simulink model "cruise_control_dut_harness"  (R2014b)
settings: Solver=FixedStepDiscrete  StartTime=0  StopTime=0.029999999999999999  FixedStep=0.01  RelTol=1e-3
undefined symbols (not defined in the file): sigbuilder_block
libraries: simulink x1
settings Model: SldvGeneratedHarnessModel=TestUnitModel=cosim_cruise_control|  RecordCoverage=on  CovMetricSettings=dcmoeb  CovHTMLOptions=-aTS=1 -bRG=1 -bTC=0 -hTR=0 -nFC=0 -scm=1 -bcm=1  covSaveCumulativeToWorkspaceVar=off  CovSaveSingleToWorkspaceVar=off  CovReportOnPause=off  CovModelRefEnable=off  CovExternalEMLEnable=on  Creator=The MathWorks Inc.  LastModifiedBy=kotsuka
settings DataIOCC: SaveFormat=StructureWithTime  SignalLoggingSaveFormat=ModelDataLogs
settings OptimizationCC: BlockReduction=off  ConditionallyExecuteInputs=off  InlineParams=on  InlineInvariantSignals=on  ExpressionFolding=off  ExpressionDepthLimit=2147483647  InitFltsAndDblsToZero=on  EfficientMapNaN2IntZero=off
settings DebuggingCC: SaveWithParameterizedLinksMsg=none  UnderspecifiedInitializationDetection=Classic  MergeDetectMultiDrivingBlocksExec=none  SignalResolutionControl=TryResolveAllWithWarning  InheritedTsInSrcMsg=none  FcnCallInpInsideContextMsg=UseLocalSettings  StateNameClashWarn=warning
settings GRTTargetCC: TargetFcnLib=ansi_tfl_tmw.mat  CombineOutputUpdateFcns=off  GRTInterface=on
settings ConfigComp: Description=Design Verifier Custom Configuration Component  DVMaxProcessTime=60  DVMakeOutputFilesUnique=off  DVParameters=on  DVModelCoverageObjectives=MCDC  DVMaxTestCaseSteps=500  DVTestSuiteOptimization=CombinedObjectives  DVAssertions=EnableAll  DVProofAssumptions=EnableAll  DVCovFilter=on  DVDetectActiveLogic=on  DVProvingStrategy=FindViolation

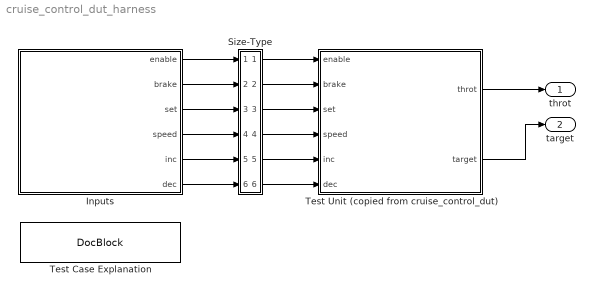
== system cruise_control_dut_harness ==
  Inputs : Subsystem  Tag=STV Subsys  LoadFcn=sigbuilder_block('load');  StartFcn=sigbuilder_block('start');  StopFcn=sigbuilder_block('stop');  ClipboardFcn=sigbuilder_block('clipboard');  mask(Sigbuilder block){}
      mask init:
      | if ~strcmp(get_param(bdroot(gcb),'SimulationStatus'),'stopped'),tuvar = sigbuilder_block('maskInit'); end
      settings: CopyFcn=sigbuilder_block('copy');  DeleteFcn=sigbuilder_block('delete');  ModelCloseFcn=sigbuilder_block('modelClose');  PreSaveFcn=sigbuilder_block('preSave');  PauseFcn=sigbuilder_block('pause');  ContinueFcn=sigbuilder_block('continue');  NameChangeFcn=sigbuilder_block('namechange');  OpenFcn=sigbuilder_block('open');  CloseFcn=sigbuilder_block('close');
      mask Display: plot(0, 0, 100, 100,[2, 2, 32, 32, 2], [68, 8, 8, 68, 68],[32, 2], [38, 38], [32, 19, 2],[53, 60, 44], [32, 17, 17, 2],[16, 16, 31, 31]);txt = getActiveGroup(gcbh);text(2, 100, txt,'verticalAlignment', 'top');
  Size-Type : Subsystem
  Test Case Explanation : simulink/Model-Wide Utilities/DocBlock  DocumentType=Text
  Test Unit (copied from cruise_control_dut) : Subsystem
  throt : Outport
  target : Outport  Port=2
  wires:
  Inputs/1(enable) -> Size-Type/1(In1)
  Size-Type/1(Out1) -> Test Unit (copied from cruise_control_dut)/1(enable)
  Inputs/2(brake) -> Size-Type/2(In2)
  Size-Type/2(Out2) -> Test Unit (copied from cruise_control_dut)/2(brake)
  Inputs/3(set) -> Size-Type/3(In3)
  Size-Type/3(Out3) -> Test Unit (copied from cruise_control_dut)/3(set)
  Inputs/4(speed) -> Size-Type/4(In4)
  Size-Type/4(Out4) -> Test Unit (copied from cruise_control_dut)/4(speed)
  Inputs/5(inc) -> Size-Type/5(In5)
  Size-Type/5(Out5) -> Test Unit (copied from cruise_control_dut)/5(inc)
  Inputs/6(dec) -> Size-Type/6(In6)
  Size-Type/6(Out6) -> Test Unit (copied from cruise_control_dut)/6(dec)
  Test Unit (copied from cruise_control_dut)/1(throt) -> throt/1
  Test Unit (copied from cruise_control_dut)/2(target) -> target/1

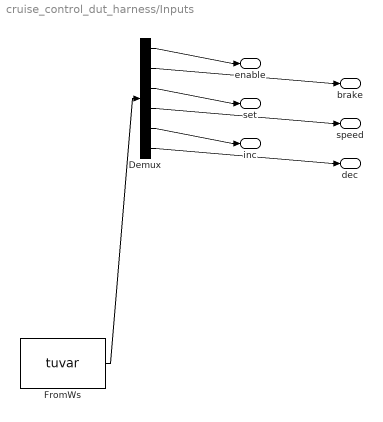
== system cruise_control_dut_harness/Inputs ==
  Demux : Demux  Tag=STV Demux  Outputs=6
  FromWs : FromWorkspace  Tag=STV FromWs  VariableName=tuvar  SampleTime=0
      SigBuilderData=|
      | dataSet(1).timeRange = [0 0.01]
      | dataSet(1).name = 'テスト ケース 1'
      | dataSet(2).timeRange = [0 0.01]
      | dataSet(2).name = 'テスト ケース 2'
      | dataSet(3).timeRange = [0 0.01]
      | dataSet(3).name = 'テスト ケース 3'
      | dataSet(4).timeRange = [0 0.01]
      | dataSet(4).name = 'テスト ケース 4'
      | dataSet(5).timeRange = [0 0.01]
      | dataSet(5).name = 'テスト ケース 5'
      | dataSet(6).timeRange = [0 0.01]
      | dataSet(6).name = 'テスト ケース 6'
      | dataSet(7).timeRange = [0 0.02]
      | dataSet(7).name = 'テスト ケース 7'
      | dataSet(8).timeRange = [0 0.03]
      | dataSet(8).name = 'テスト ケース 8'
      | dataSet(9).timeRange = [0 0.03]
      | dataSet(9).name = 'テスト ケース 9'
      | sbobj.Name = 'Signal Builder'
      | sbobj.Groups(1).Name = 'テスト ケース 1'
      | sbobj.Groups(1).Signals(1).Name = 'enable'
      | sbobj.Groups(1).Signals(1).XData = [0 0.01]
      | sbobj.Groups(1).Signals(1).YData = [0 0]
      | sbobj.Groups(1).Signals(2).Name = 'brake'
      | sbobj.Groups(1).Signals(2).XData = [0 0.01]
      | sbobj.Groups(1).Signals(2).YData = [0 0]
      | sbobj.Groups(1).Signals(3).Name = 'set'
      | sbobj.Groups(1).Signals(3).XData = [0 0.01]
      | sbobj.Groups(1).Signals(3).YData = [1 1]
      | sbobj.Groups(1).Signals(4).Name = 'speed'
      | sbobj.Groups(1).Signals(4).XData = [0 0.01]
      | sbobj.Groups(1).Signals(4).YData = [0 0]
      | sbobj.Groups(1).Signals(5).Name = 'inc'
      | sbobj.Groups(1).Signals(5).XData = [0 0.01]
      | sbobj.Groups(1).Signals(5).YData = [0 0]
      | sbobj.Groups(1).Signals(6).Name = 'dec'
      | sbobj.Groups(1).Signals(6).XData = [0 0.01]
      | sbobj.Groups(1).Signals(6).YData = [0 0]
      | sbobj.Groups(1).TimeRange = [0 0.01]
      | sbobj.Groups(2).Name = 'テスト ケース 2'
      | sbobj.Groups(2).Signals(1).Name = 'enable'
      | sbobj.Groups(2).Signals(1).XData = [0 0.01]
      | sbobj.Groups(2).Signals(1).YData = [1 1]
      | sbobj.Groups(2).Signals(2).Name = 'brake'
      | sbobj.Groups(2).Signals(2).XData = [0 0.01]
      | sbobj.Groups(2).Signals(2).YData = [1 1]
      | sbobj.Groups(2).Signals(3).Name = 'set'
      | sbobj.Groups(2).Signals(3).XData = [0 0.01]
      | sbobj.Groups(2).Signals(3).YData = [1 1]
      | sbobj.Groups(2).Signals(4).Name = 'speed'
      | sbobj.Groups(2).Signals(4).XData = [0 0.01]
      | sbobj.Groups(2).Signals(4).YData = [0 0]
      | sbobj.Groups(2).Signals(5).Name = 'inc'
      | sbobj.Groups(2).Signals(5).XData = [0 0.01]
      | sbobj.Groups(2).Signals(5).YData = [0 0]
      | sbobj.Groups(2).Signals(6).Name = 'dec'
      | sbobj.Groups(2).Signals(6).XData = [0 0.01]
      | sbobj.Groups(2).Signals(6).YData = [0 0]
      | sbobj.Groups(2).TimeRange = [0 0.01]
      | sbobj.Groups(3).Name = 'テスト ケース 3'
      | sbobj.Groups(3).Signals(1).Name = 'enable'
      | sbobj.Groups(3).Signals(1).XData = [0 0.01]
      | sbobj.Groups(3).Signals(1).YData = [0 0]
      | sbobj.Groups(3).Signals(2).Name = 'brake'
      | sbobj.Groups(3).Signals(2).XData = [0 0.01]
      | sbobj.Groups(3).Signals(2).YData = [0 0]
      | sbobj.Groups(3).Signals(3).Name = 'set'
      | sbobj.Groups(3).Signals(3).XData = [0 0.01]
      | sbobj.Groups(3).Signals(3).YData = [0 0]
      | sbobj.Groups(3).Signals(4).Name = 'speed'
      | sbobj.Groups(3).Signals(4).XData = [0 0.01]
      | sbobj.Groups(3).Signals(4).YData = [0 0]
      | sbobj.Groups(3).Signals(5).Name = 'inc'
      | sbobj.Groups(3).Signals(5).XData = [0 0.01]
      | sbobj.Groups(3).Signals(5).YData = [1 1]
      | sbobj.Groups(3).Signals(6).Name = 'dec'
      | sbobj.Groups(3).Signals(6).XData = [0 0.01]
      | sbobj.Groups(3).Signals(6).YData = [0 0]
      | sbobj.Groups(3).TimeRange = [0 0.01]
      | sbobj.Groups(4).Name = 'テスト ケース 4'
      | sbobj.Groups(4).Signals(1).Name = 'enable'
      | sbobj.Groups(4).Signals(1).XData = [0 0.01]
      | sbobj.Groups(4).Signals(1).YData = [1 1]
      | sbobj.Groups(4).Signals(2).Name = 'brake'
      | sbobj.Groups(4).Signals(2).XData = [0 0.01]
      | sbobj.Groups(4).Signals(2).YData = [0 0]
      | sbobj.Groups(4).Signals(3).Name = 'set'
      | sbobj.Groups(4).Signals(3).XData = [0 0.01]
      | sbobj.Groups(4).Signals(3).YData = [0 0]
      | sbobj.Groups(4).Signals(4).Name = 'speed'
      | sbobj.Groups(4).Signals(4).XData = [0 0.01]
      | sbobj.Groups(4).Signals(4).YData = [0 0]
      | sbobj.Groups(4).Signals(5).Name = 'inc'
      | sbobj.Groups(4).Signals(5).XData = [0 0.01]
      | sbobj.Groups(4).Signals(5).YData = [1 1]
      | sbobj.Groups(4).Signals(6).Name = 'dec'
      | sbobj.Groups(4).Signals(6).XData = [0 0.01]
      | sbobj.Groups(4).Signals(6).YData = [0 0]
      | sbobj.Groups(4).TimeRange = [0 0.01]
      | sbobj.Groups(5).Name = 'テスト ケース 5'
      | sbobj.Groups(5).Signals(1).Name = 'enable'
      | sbobj.Groups(5).Signals(1).XData = [0 0.01]
      | sbobj.Groups(5).Signals(1).YData = [1 1]
      | sbobj.Groups(5).Signals(2).Name = 'brake'
      | sbobj.Groups(5).Signals(2).XData = [0 0.01]
      | sbobj.Groups(5).Signals(2).YData = [0 0]
      | sbobj.Groups(5).Signals(3).Name = 'set'
      | sbobj.Groups(5).Signals(3).XData = [0 0.01]
      | sbobj.Groups(5).Signals(3).YData = [1 1]
      | sbobj.Groups(5).Signals(4).Name = 'speed'
      | sbobj.Groups(5).Signals(4).XData = [0 0.01]
      | sbobj.Groups(5).Signals(4).YData = [0 0]
      | sbobj.Groups(5).Signals(5).Name = 'inc'
      | sbobj.Groups(5).Signals(5).XData = [0 0.01]
      | sbobj.Groups(5).Signals(5).YData = [0 0]
      | sbobj.Groups(5).Signals(6).Name = 'dec'
      | sbobj.Groups(5).Signals(6).XData = [0 0.01]
      | sbobj.Groups(5).Signals(6).YData = [0 0]
      | sbobj.Groups(5).TimeRange = [0 0.01]
      | sbobj.Groups(6).Name = 'テスト ケース 6'
      | sbobj.Groups(6).Signals(1).Name = 'enable'
      | sbobj.Groups(6).Signals(1).XData = [0 0.01]
      | sbobj.Groups(6).Signals(1).YData = [0 0]
      | sbobj.Groups(6).Signals(2).Name = 'brake'
      | sbobj.Groups(6).Signals(2).XData = [0 0.01]
      | sbobj.Groups(6).Signals(2).YData = [0 0]
      | sbobj.Groups(6).Signals(3).Name = 'set'
      | sbobj.Groups(6).Signals(3).XData = [0 0.01]
      | sbobj.Groups(6).Signals(3).YData = [1 1]
      | sbobj.Groups(6).Signals(4).Name = 'speed'
      | sbobj.Groups(6).Signals(4).XData = [0 0.01]
      | sbobj.Groups(6).Signals(4).YData = [0 0]
      | sbobj.Groups(6).Signals(5).Name = 'inc'
      | sbobj.Groups(6).Signals(5).XData = [0 0.01]
      | sbobj.Groups(6).Signals(5).YData = [0 0]
      | sbobj.Groups(6).Signals(6).Name = 'dec'
      | sbobj.Groups(6).Signals(6).XData = [0 0.01]
      | sbobj.Groups(6).Signals(6).YData = [1 1]
      | sbobj.Groups(6).TimeRange = [0 0.01]
      | sbobj.Groups(7).Name = 'テスト ケース 7'
      | sbobj.Groups(7).Signals(1).Name = 'enable'
      | sbobj.Groups(7).Signals(1).XData = [0 0.01 0.02]
      | sbobj.Groups(7).Signals(1).YData = [1 1 1]
      | sbobj.Groups(7).Signals(2).Name = 'brake'
      | sbobj.Groups(7).Signals(2).XData = [0 0.01 0.02]
      | sbobj.Groups(7).Signals(2).YData = [0 0 0]
      | sbobj.Groups(7).Signals(3).Name = 'set'
      | sbobj.Groups(7).Signals(3).XData = [0 0.01 0.01 0.02]
      | sbobj.Groups(7).Signals(3).YData = [1 1 0 0]
      | sbobj.Groups(7).Signals(4).Name = 'speed'
      | sbobj.Groups(7).Signals(4).XData = [0 0.01 0.02]
      | sbobj.Groups(7).Signals(4).YData = [0 0 0]
      | sbobj.Groups(7).Signals(5).Name = 'inc'
      | sbobj.Groups(7).Signals(5).XData = [0 0.01 0.01 0.02]
      | sbobj.Groups(7).Signals(5).YData = [1 1 0 0]
      | sbobj.Groups(7).Signals(6).Name = 'dec'
      | sbobj.Groups(7).Signals(6).XData = [0 0.01 0.02]
      | sbobj.Groups(7).Signals(6).YData = [0 0 0]
      | sbobj.Groups(7).TimeRange = [0 0.02]
      | sbobj.Groups(8).Name = 'テスト ケース 8'
      | sbobj.Groups(8).Signals(1).Name = 'enable'
      | sbobj.Groups(8).Signals(1).XData = [0 0.01 0.02 0.03]
      | sbobj.Groups(8).Signals(1).YData = [1 1 1 1]
      | sbobj.Groups(8).Signals(2).Name = 'brake'
      | sbobj.Groups(8).Signals(2).XData = [0 0.01 0.02 0.03]
      | sbobj.Groups(8).Signals(2).YData = [0 0 0 0]
      | sbobj.Groups(8).Signals(3).Name = 'set'
      | sbobj.Groups(8).Signals(3).XData = [0 0.01 0.01 0.02 0.02 0.03]
      | sbobj.Groups(8).Signals(3).YData = [1 1 0 0 1 1]
      | sbobj.Groups(8).Signals(4).Name = 'speed'
      | sbobj.Groups(8).Signals(4).XData = [0 0.01 0.01 0.02 0.02 0.03]
      | sbobj.Groups(8).Signals(4).YData = [0 0 -499 -499 0 0]
      | sbobj.Groups(8).Signals(5).Name = 'inc'
      | sbobj.Groups(8).Signals(5).XData = [0 0.01 0.02 0.02 0.03]
      | sbobj.Groups(8).Signals(5).YData = [1 1 1 0 0]
      | sbobj.Groups(8).Signals(6).Name = 'dec'
      | sbobj.Groups(8).Signals(6).XData = [0 0.01 0.02 0.03]
      | sbobj.Groups(8).Signals(6).YData = [0 0 0 0]
      | sbobj.Groups(8).TimeRange = [0 0.03]
      | sbobj.Groups(9).Name = 'テスト ケース 9'
      | sbobj.Groups(9).Signals(1).Name = 'enable'
      | sbobj.Groups(9).Signals(1).XData = [0 0.01 0.02 0.03]
      | sbobj.Groups(9).Signals(1).YData = [1 1 1 1]
      | sbobj.Groups(9).Signals(2).Name = 'brake'
      | sbobj.Groups(9).Signals(2).XData = [0 0.01 0.02 0.03]
      | sbobj.Groups(9).Signals(2).YData = [0 0 0 0]
      | sbobj.Groups(9).Signals(3).Name = 'set'
      | sbobj.Groups(9).Signals(3).XData = [0 0.01 0.01 0.02 0.02 0.03]
      | sbobj.Groups(9).Signals(3).YData = [1 1 0 0 1 1]
      | sbobj.Groups(9).Signals(4).Name = 'speed'
      | sbobj.Groups(9).Signals(4).XData = [0 0.01 0.01 0.02 0.02 0.03]
      | sbobj.Groups(9).Signals(4).YData = [0 0 501 501 0 0]
      | sbobj.Groups(9).Signals(5).Name = 'inc'
      | sbobj.Groups(9).Signals(5).XData = [0 0.01 0.02 0.02 0.03]
      | sbobj.Groups(9).Signals(5).YData = [1 1 1 0 0]
      | sbobj.Groups(9).Signals(6).Name = 'dec'
      | sbobj.Groups(9).Signals(6).XData = [0 0.01 0.02 0.03]
      | sbobj.Groups(9).Signals(6).YData = [0 0 0 0]
      | sbobj.Groups(9).TimeRange = [0 0.03]
  enable : Outport  Tag=STV Outport
  brake : Outport  Tag=STV Outport  Port=2
  set : Outport  Tag=STV Outport  Port=3
  speed : Outport  Tag=STV Outport  Port=4
  inc : Outport  Tag=STV Outport  Port=5
  dec : Outport  Tag=STV Outport  Port=6
  wires:
  FromWs/1 -> Demux/1
  Demux/1 -> enable/1
  Demux/2 -> brake/1
  Demux/3 -> set/1
  Demux/4 -> speed/1
  Demux/5 -> inc/1
  Demux/6 -> dec/1

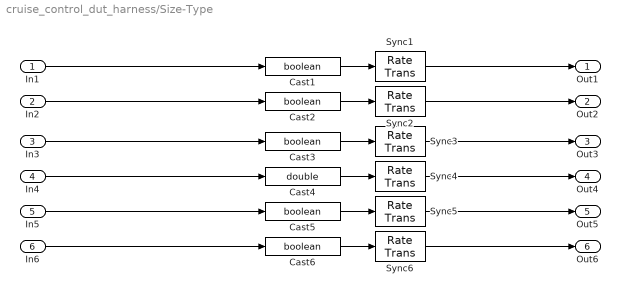
== system cruise_control_dut_harness/Size-Type ==
  In1 : Inport
  In2 : Inport  Port=2
  In3 : Inport  Port=3
  In4 : Inport  Port=4
  In5 : Inport  Port=5
  In6 : Inport  Port=6
  Cast{1..3,5..6} (5 alike) : DataTypeConversion  OutDataTypeStr=boolean  RndMeth=Nearest  SaturateOnIntegerOverflow=on
  Cast4 : DataTypeConversion  OutDataTypeStr=double  RndMeth=Nearest  SaturateOnIntegerOverflow=on
  Sync{1..6} (6 alike) : RateTransition  OutPortSampleTime=[0.01,0]
  Out1 : Outport
  Out2 : Outport  Port=2
  Out3 : Outport  Port=3
  Out4 : Outport  Port=4
  Out5 : Outport  Port=5
  Out6 : Outport  Port=6
  wires:
  In1/1 -> Cast1/1
  Cast1/1 -> Sync1/1
  Sync1/1 -> Out1/1
  In2/1 -> Cast2/1
  Cast2/1 -> Sync2/1
  Sync2/1 -> Out2/1
  In3/1 -> Cast3/1
  Cast3/1 -> Sync3/1
  Sync3/1 -> Out3/1
  In4/1 -> Cast4/1
  Cast4/1 -> Sync4/1
  Sync4/1 -> Out4/1
  In5/1 -> Cast5/1
  Cast5/1 -> Sync5/1
  Sync5/1 -> Out5/1
  In6/1 -> Cast6/1
  Cast6/1 -> Sync6/1
  Sync6/1 -> Out6/1

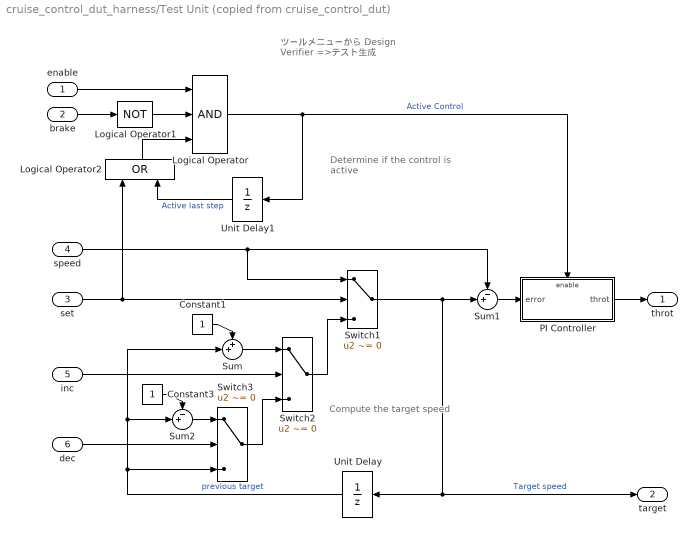
== system cruise_control_dut_harness/Test Unit (copied from cruise_control_dut) ==
  note: Compute the
      | target speed
  note: Determine if the
      | control is active
  note: ツールメニューから
      | Design Verifier
      | =>テスト生成
  enable : Inport  OutDataTypeStr=boolean
  brake : Inport  Port=2  OutDataTypeStr=boolean
  set : Inport  Port=3  OutDataTypeStr=boolean
  speed : Inport  Port=4  OutDataTypeStr=double
  inc : Inport  Port=5  OutDataTypeStr=boolean
  dec : Inport  Port=6  OutDataTypeStr=boolean
  Constant1 : Constant
  Constant3 : Constant
  Logical Operator : Logic  Inputs=3  AllPortsSameDT=off  OutDataTypeStr=boolean
  Logical Operator1 : Logic  Operator=NOT  AllPortsSameDT=off  OutDataTypeStr=boolean
  Logical Operator2 : Logic  Operator=OR  AllPortsSameDT=off  OutDataTypeStr=boolean
  PI Controller : Subsystem
  Sum : Sum  Inputs=++|
  Sum1 : Sum  Inputs=-+|
  Sum2 : Sum  Inputs=-+|
  Switch1 : Switch  Criteria=u2 ~= 0
  Switch2 : Switch  Criteria=u2 ~= 0
  Switch3 : Switch  Criteria=u2 ~= 0
  Unit Delay : UnitDelay  SampleTime=0.01
  Unit Delay1 : UnitDelay  SampleTime=0.01
  throt : Outport
  target : Outport  Port=2
  wires:
  PI Controller/1(throt) -> throt/1
  Sum1/1 -> PI Controller/1(error)
  Logical Operator/1 -> Unit Delay1/1, PI Controller/Enable  "Active Control"
  Unit Delay1/1 -> Logical Operator2/2  "Active last step"
  Logical Operator2/1 -> Logical Operator/3
  Switch1/1 -> Unit Delay/1, target/1, Sum1/2  "Target speed"
  Unit Delay/1 -> Sum/2, Sum2/2, Switch3/3  "previous target"
  Switch3/1 -> Switch2/3
  Switch2/1 -> Switch1/3
  Sum2/1 -> Switch3/1
  Constant3/1 -> Sum2/1
  dec/1 -> Switch3/2
  Sum/1 -> Switch2/1
  Constant1/1 -> Sum/1
  inc/1 -> Switch2/2
  speed/1 -> Sum1/1, Switch1/1
  set/1 -> Switch1/2, Logical Operator2/1
  Logical Operator1/1 -> Logical Operator/2
  enable/1 -> Logical Operator/1
  brake/1 -> Logical Operator1/1

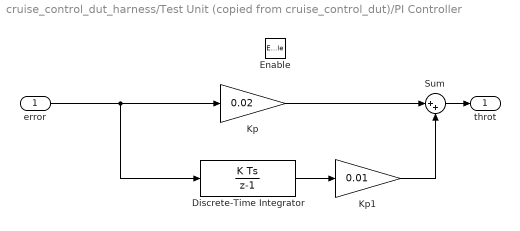
== system cruise_control_dut_harness/Test Unit (copied from cruise_control_dut)/PI Controller ==
  error : Inport
  Enable : EnablePort
  Discrete-Time Integrator : DiscreteIntegrator  SampleTime=0.01  LimitOutput=on  UpperSaturationLimit=5  LowerSaturationLimit=-5
  Kp : Gain  Gain=0.02
  Kp1 : Gain  Gain=0.01
  Sum : Sum  Inputs=|++
  throt : Outport  InitialOutput=0
  wires:
  Kp/1 -> Sum/1
  Kp1/1 -> Sum/2
  Discrete-Time Integrator/1 -> Kp1/1
  error/1 -> Kp/1, Discrete-Time Integrator/1
  Sum/1 -> throt/1
